simulink subsystem "PieroAdryZ"  (R2023b)
settings: Solver=VariableStepAuto  StartTime=0.0  StopTime=10.0  RelTol=1e-3
settings Model: Creator=adria  LastModifiedBy=adria

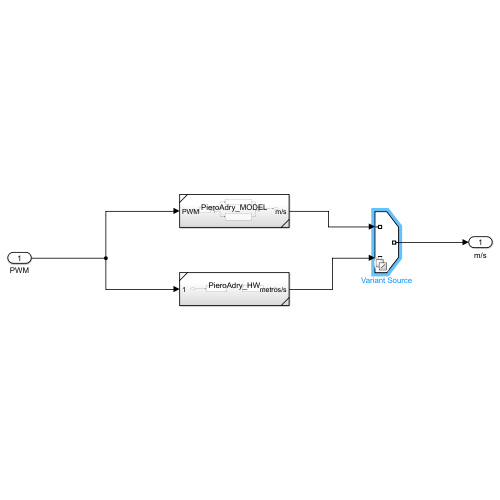
[thumbnail: Simulink's stored preview of the top-level diagram]
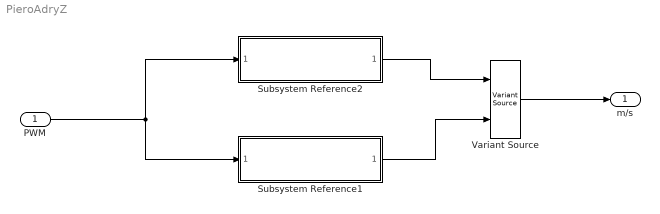
== system PieroAdryZ ==
  PWM : Inport
  Subsystem Reference1 : Subsystem  ReferencedSubsystem=PieroAdry_HW
  Subsystem Reference2 : Subsystem  ReferencedSubsystem=PieroAdry_MODELZ
  Variant Source : VariantSource  VariantControlMode=sim codegen switching
  m/s : Outport
  wires:
  PWM/1 -> Subsystem Reference1/1, Subsystem Reference2/1
  Subsystem Reference2/1 -> Variant Source/1
  Subsystem Reference1/1 -> Variant Source/2
  Variant Source/1 -> m/s/1
